simulink model "Example_IOBlock_Library_EEPROM_Offset_Access"  (Simulink 10.3)
settings: Solver=FixedStepDiscrete  StartTime=0.0  StopTime=10.0  FixedStep=0.01  RelTol=1e-3
PreLoadFcn:
  | DERATE_PRINTF = 20;
libraries: IOBlock_Library_TTC580 x23, simulink x4
(part 2 of 2)

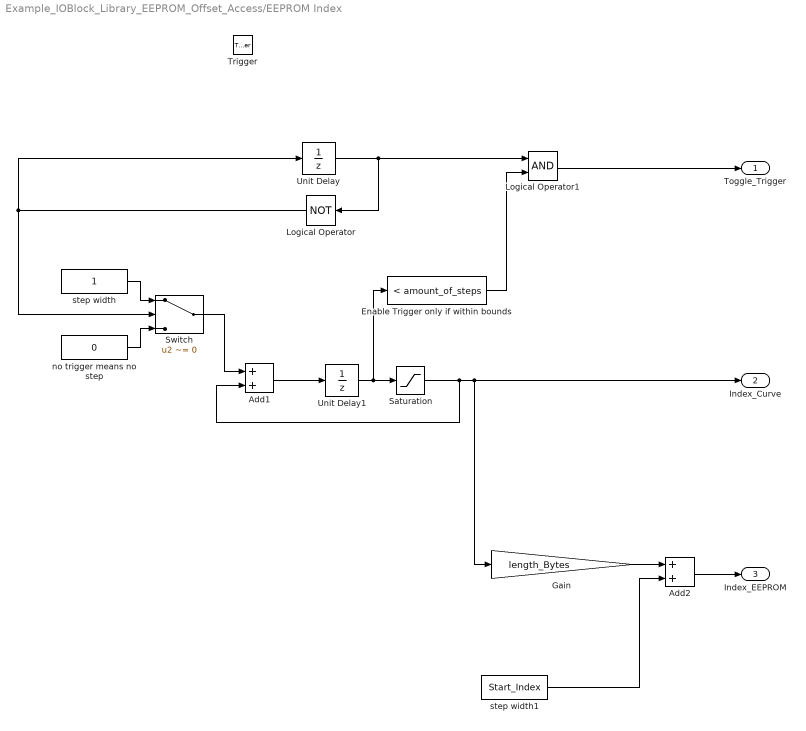
== system Example_IOBlock_Library_EEPROM_Offset_Access/EEPROM Index   ==
  Trigger : TriggerPort  TriggerType=either  VariantControl=(inherit)  PortDimensions=1
  Add1 : Sum  SaturateOnIntegerOverflow=on
  Add2 : Sum  SaturateOnIntegerOverflow=on
  Enable Trigger only if within bounds : simulink/Logic and Bit Operations/Compare To Constant  relop=<  const=amount_of_steps  OutDataTypeStr=boolean
  Gain : Gain  Gain=length_Bytes  OutDataTypeStr=uint16
  Logical Operator : Logic  Operator=NOT  AllPortsSameDT=off  OutDataTypeStr=boolean
  Logical Operator1 : Logic  AllPortsSameDT=off  OutDataTypeStr=boolean
  Saturation : Saturate  UpperLimit=(amount_of_steps-1); %zero based  LowerLimit=0
  Switch : Switch  Criteria=u2 ~= 0
  Unit Delay : UnitDelay  InitialCondition=1  SampleTime=-1  HasFrameUpgradeWarning=on
  Unit Delay1 : UnitDelay  SampleTime=-1  HasFrameUpgradeWarning=on
  no trigger means no step : Constant  Value=0  OutDataTypeStr=uint16
  step width : Constant  OutDataTypeStr=uint16
  step width1 : Constant  Value=Start_Index  OutDataTypeStr=uint16
  Toggle_Trigger : Outport  OutDataTypeStr=boolean  InitialOutput=0  VectorParamsAs1DForOutWhenUnconnected=off
  Index_Curve : Outport  Port=2  PortDimensions=1  VectorParamsAs1DForOutWhenUnconnected=off
  Index_EEPROM : Outport  Port=3  PortDimensions=1  InitialOutput=Start_Index  VectorParamsAs1DForOutWhenUnconnected=off
  wires:
  Logical Operator/1 -> Switch/2, Unit Delay/1
  Unit Delay/1 -> Logical Operator/1, Logical Operator1/1
  Unit Delay1/1 -> Enable Trigger only if within bounds/1, Saturation/1
  Add1/1 -> Unit Delay1/1
  Saturation/1 -> Add1/2, Gain/1, Index_Curve/1
  Enable Trigger only if within bounds/1 -> Logical Operator1/2
  Logical Operator1/1 -> Toggle_Trigger/1
  Switch/1 -> Add1/1
  step width/1 -> Switch/1
  no trigger means no step/1 -> Switch/3
  Gain/1 -> Add2/1
  step width1/1 -> Add2/2
  Add2/1 -> Index_EEPROM/1

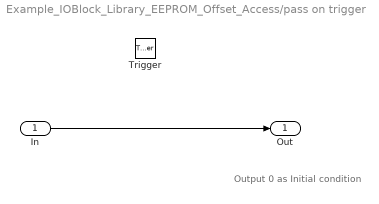
== system Example_IOBlock_Library_EEPROM_Offset_Access/pass on trigger ==
  note: Output 0 as Initial condition
  In : Inport
  Trigger : TriggerPort  VariantControl=(inherit)
  Out : Outport  InitialOutput=0  VectorParamsAs1DForOutWhenUnconnected=off
  wires:
  In/1 -> Out/1

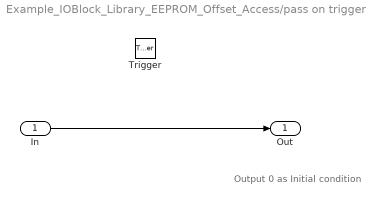
== system Example_IOBlock_Library_EEPROM_Offset_Access/pass on trigger  ==
  note: Output 0 as Initial condition
  In : Inport
  Trigger : TriggerPort  VariantControl=(inherit)
  Out : Outport  InitialOutput=0  VectorParamsAs1DForOutWhenUnconnected=off
  wires:
  In/1 -> Out/1
